simulink library "fva"  (Simulink 8.1)
settings: Solver=ode1  StartTime=0.0  StopTime=Inf  FixedStep=0.001  RelTol=1e-3
PostLoadFcn:
  | , if any(exist('dsrtsu_mdlpostloadfcn', 'file') == [2, 3, 6]), try dsrtsu_mdlpostloadfcn('Execute', bdroot); catch fprintf('Error in PostLoadFcn (dsrtsu_mdlpostloadfcn) for model "%s":\n %s\n', bdroot, lasterr); end, end,
undefined symbols (not defined in the file or in its folder): FALSE, TRUE
settings Model: DSRTSU_INTERNAL_RTI_VER=450  DSRTSU_INTERNAL_RTI_TYPE=rti1401  RTICANMMDATA=struct('GeneralSetupData',struct('modelroot','D:\ELN150201_TAIWAN\trunk\AdasDragon\software\sw_development\arch\app\jud','generalsettings',struct('filesettings',struct('destfolder',struct('Name','RTICANMM_FILES','Check',1),'buildfolder',struct('Name','.','Check',1),'AbsDestfolder',struct('Name','D:\ELN150201_TAIWAN\trunk\AdasDragon\software\sw_development\arch\app\jud\RTICANMM_FILES'),'AbsBuildfolder',struct('Name','D:\ELN150201_TAIWAN\trunk\AdasDragon\software\sw_development\arch\app\jud'))),'options',struct('addpaths',1,'rmpaths',1,'addtrcexclusion',logical(1),'cannavigator',struct('checkmonitoring',0),'show_usrtrc',0,'use_usrtrc',0),'advanced',struct('options',[1 1 1 1 1 1 1 1 1 1 1 1 1 1 1 1 1 1 1 1 1 1 1 1 1 1 1 1 1 1 1 1 1 1 1 1 1 1 1 1 1 1 1 1 1 1 1 1 1 1 1 1 1 1 1 1 1 1 1 1 1 1 1 1 1 1 1 1 1 1 1 1 1 1 1 1 1 1 1 1 1 1 1 1 1 1 1 1 1 1 1 1 1 1 1 1 1 1 1 1]),'MPSetup',{{}},'modelname','fva','block','fva'))  DSRTSU_INTERNAL_RTIFPGA=40  Creator=tescamilla  LastModifiedBy=AT015555

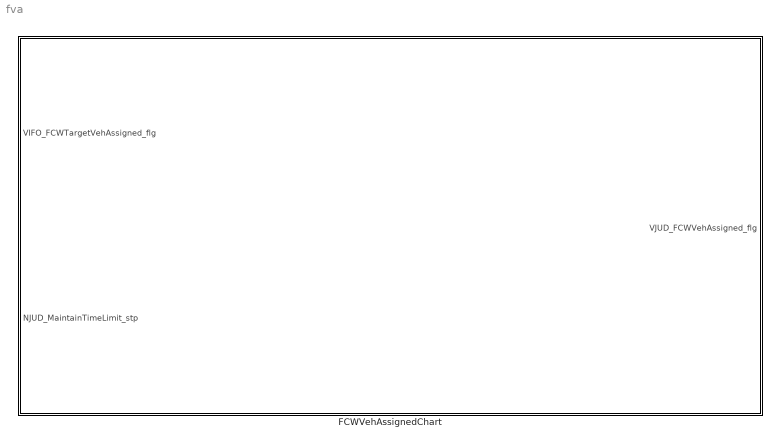
== system fva ==
  FCWVehAssignedChart : Stateflow chart  TreatAsAtomicUnit=on

== stateflow chart FCWVehAssignedChart ==
  state VEH_NOT_ASSIGNED
    en:
    VJUD_FCWVehAssigned_flg = FALSE;
  state VEH_ASSIGNED
    en:
    VJUD_FCWVehAssigned_flg = TRUE;
  state MAINTAIN
    en:
    NJUD_MaintainTimeLocal_stp = 0;
    du:
    NJUD_MaintainTimeLocal_stp=NJUD_MaintainTimeLocal_stp+1;
  (default) -> VEH_NOT_ASSIGNED
  (junction 12) -> VEH_NOT_ASSIGNED : [NJUD_MaintainTimeLocal_stp>NJUD_MaintainTimeLimit_stp...
      | && VIFO_FCWTargetVehAssigned_flg ==FALSE]
  MAINTAIN -> (junction 12) [order 2]
  VEH_NOT_ASSIGNED -> (junction 13)
  VEH_ASSIGNED -> MAINTAIN : [VIFO_FCWTargetVehAssigned_flg==FALSE]
  (junction 13) -> VEH_ASSIGNED : [VIFO_FCWTargetVehAssigned_flg==TRUE]
  MAINTAIN -> VEH_ASSIGNED [order 1] : [VIFO_FCWTargetVehAssigned_flg ==TRUE]
  data: VJUD_FCWVehAssigned_flg output boolean; VIFO_FCWTargetVehAssigned_flg input boolean; FALSE parameter double; TRUE parameter double; NJUD_MaintainTimeLocal_stp local single; NJUD_MaintainTimeLimit_stp input single
